simulink model "VCU_Modes"  (R2025b)
settings: Solver=FixedStepDiscrete  StartTime=0.0  StopTime=10.0  FixedStep=0.01  RelTol=1e-3
values from neighbouring files (symbols this model uses):
  c_VCU_BattCurrDrvThd = 100.0    [VCU_Modes.sldd]
  c_VCU_BattCurrDrvTime = 200.0    [VCU_Modes.sldd]
  c_VCU_BattCurrParkThd = 5.0    [VCU_Modes.sldd]
  c_VCU_BattCurrPeakDrvThd = 180.0    [VCU_Modes.sldd]
  c_VCU_BattSocDrvThd = 10.0    [VCU_Modes.sldd]
  c_VCU_BattSocLimpThd = 5.0    [VCU_Modes.sldd]
  c_VCU_BattTempDrvThdMax = 60.0    [VCU_Modes.sldd]
  c_VCU_BattTempParkThd = 45.0    [VCU_Modes.sldd]
  c_VCU_BattTempParkThdFlt = 55.0    [VCU_Modes.sldd]
  c_VCU_DrvThdWait = 100.0    [VCU_Modes.sldd]
  c_VCU_EcuTempDrvThdMax = 95.0    [VCU_Modes.sldd]
  c_VCU_EcuTempParkThd = 70.0    [VCU_Modes.sldd]
  c_VCU_EcuTempParkThdFlt = 85.0    [VCU_Modes.sldd]
  c_VCU_FailSafeThdTime = 200.0    [VCU_Modes.sldd]
  c_VCU_FrontLampExclusive_B = 0.0    [VCU_Modes.sldd]
  c_VCU_HeadLampAmbientThd = 300.0    [VCU_Modes.sldd]
  c_VCU_HeadlampAutoEnable_B = 1.0    [VCU_Modes.sldd]
  c_VCU_HeadlampManualOverride_B = 1.0    [VCU_Modes.sldd]
  c_VCU_LongPressTimeThd = 200.0    [VCU_Modes.sldd]
  c_VCU_MotTempDrvThdMax = 120.0    [VCU_Modes.sldd]
  c_VCU_MotTempParkThd = 80.0    [VCU_Modes.sldd]
  c_VCU_MotTempParkThdFlt = 100.0    [VCU_Modes.sldd]
  c_VCU_ParkExtThdWait = 100.0    [VCU_Modes.sldd]
  c_VCU_ParkThdWait = 100.0    [VCU_Modes.sldd]
  F32_ZERO = 0.0    [VCU_Modes.sldd]
  FALSE = 0.0    [VCU_Modes.sldd]
  TRUE = 1.0    [VCU_Modes.sldd]
  UI8_ZERO = 0.0    [VCU_Modes.sldd]
undefined symbols (not defined in the file or in its folder): POWER_MODE, SIG_STATUS, VCU_MODE
libraries: Sanu_Lib x9, simulink x1
(part 1 of 2)
Description:
  | Different types of VCU modes and Drive modes control.
  | Based on VCU and Drive modes vehicle performance.
settings Model: DataDictionary=VCU_Modes.sldd  Creator=2503-00091  LastModifiedBy=2503-00091
settings OptimizationCC: DefaultParameterBehavior=Inlined  EnhancedBackFolding=on  PassReuseOutputArgsAs=Individual arguments  ZeroExternalMemoryAtStartup=off  ZeroInternalMemoryAtStartup=off  OptimizeBlockOrder=speed  DifferentSizesBufferReuse=on  OptimizationCustomize=off  LabelGuidedReuse=on  EfficientTunableParamExpr=on
settings DebuggingCC: AlgebraicLoopMsg=error  ArtificialAlgebraicLoopMsg=error  ParameterTunabilityLossMsg=error  UnitsInconsistencyMsg=none
settings SFSimCC: MATLABDynamicMemAlloc=off
settings RTWCC: SystemTargetFile=ert.tlc  TemplateMakefile=ert_default_tmf  Description=Embedded Coder
settings CodeAppCC: ForceParamTrailComments=on  IgnoreCustomStorageClasses=off  OperatorAnnotations=on  SimulinkDataObjDesc=on  SFDataObjDesc=on  MATLABFcnDesc=on  CustomSymbolStrFcnArg=$I$N$M  CustomSymbolStrBlkIO=$N$M  InsertBlockDesc=on
settings ERTTargetCC: ERTCustomFileTemplate=example_file_process.tlc  TargetLangStandard=C99 (ISO)  GenerateSampleERTMain=on  LogVarNameModifier=none

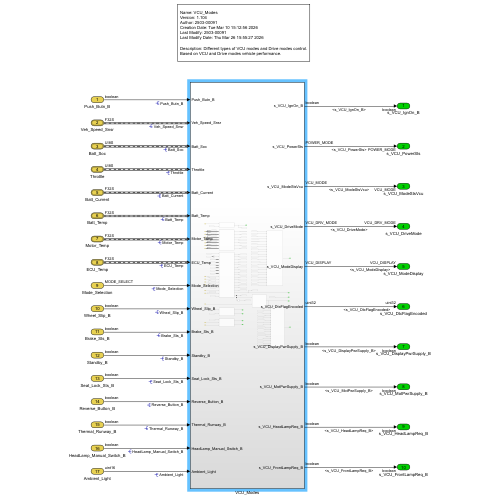
[thumbnail: Simulink's stored preview of the top-level diagram]
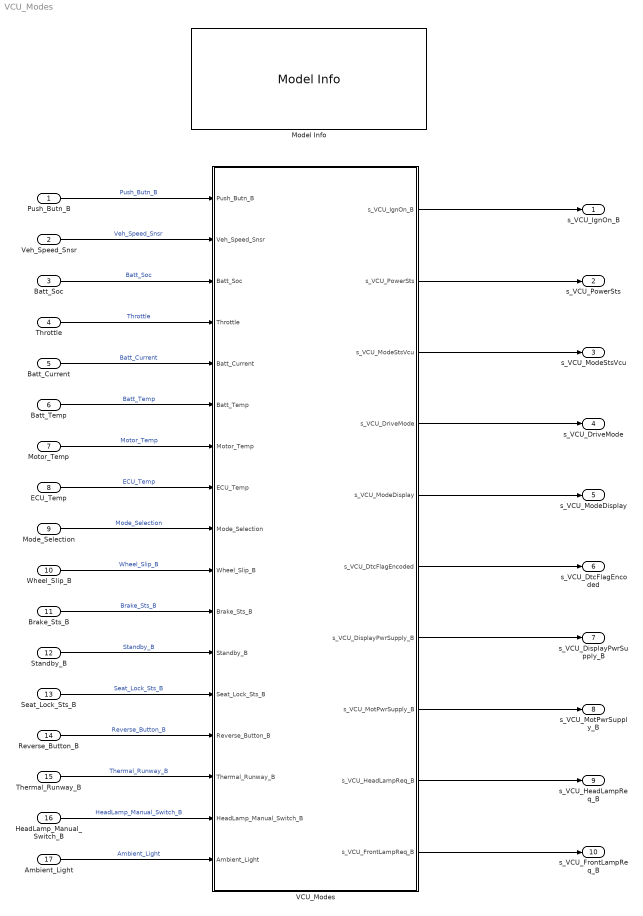
== system VCU_Modes ==
  Push_Butn_B : Inport  OutDataTypeStr=boolean  PortDimensions=1
  Veh_Speed_Snsr : Inport  Port=2  OutDataTypeStr=Bus: F32S  PortDimensions=1  BusOutputAsStruct=on
  Batt_Soc : Inport  Port=3  OutDataTypeStr=Bus: UI8S  PortDimensions=1  BusOutputAsStruct=on
  Throttle : Inport  Port=4  OutDataTypeStr=Bus: UI8S  PortDimensions=1  BusOutputAsStruct=on
  Batt_Current : Inport  Port=5  OutDataTypeStr=Bus: F32S  PortDimensions=1  BusOutputAsStruct=on
  Batt_Temp : Inport  Port=6  OutDataTypeStr=Bus: F32S  PortDimensions=1  BusOutputAsStruct=on
  Motor_Temp : Inport  Port=7  OutDataTypeStr=Bus: F32S  PortDimensions=1  BusOutputAsStruct=on
  ECU_Temp : Inport  Port=8  OutDataTypeStr=Bus: F32S  PortDimensions=1  BusOutputAsStruct=on
  Mode_Selection : Inport  Port=9  OutDataTypeStr=Enum: MODE_SELECT  PortDimensions=1
  Wheel_Slip_B : Inport  Port=10  OutDataTypeStr=boolean  PortDimensions=1
  Brake_Sts_B : Inport  Port=11  OutDataTypeStr=boolean  PortDimensions=1
  Standby_B : Inport  Port=12  OutDataTypeStr=boolean  PortDimensions=1
  Seat_Lock_Sts_B : Inport  Port=13  OutDataTypeStr=boolean  PortDimensions=1
  Reverse_Button_B : Inport  Port=14  OutDataTypeStr=boolean  PortDimensions=1
  Thermal_Runway_B : Inport  Port=15  OutDataTypeStr=boolean  PortDimensions=1
  HeadLamp_Manual_Switch_B : Inport  Port=16  OutDataTypeStr=boolean  PortDimensions=1
  Ambient_Light : Inport  Port=17  OutDataTypeStr=uint16  PortDimensions=1
  Model Info : simulink/Model-Wide Utilities/Model Info  Frame=on  DisplayStringWithTags=|  HorizontalTextAlignment=Left  LeftAlignmentValue=0.02
      | Name: %<ModelName>
      | Version: %<ModelVersion>
      | Author: %<Creator>
      | Creation Date: %<Created>
      | Last Modify: %<LastModifiedBy>
      | Last Modify Date: %<LastModificationDate>
      | 
      | Description: %<Description>
  VCU_Modes : Subsystem
  s_VCU_IgnOn_B : Outport  OutDataTypeStr=boolean  PortDimensions=1
  s_VCU_PowerSts : Outport  Port=2  OutDataTypeStr=Enum: POWER_MODE  PortDimensions=1
  s_VCU_ModeStsVcu : Outport  Port=3  OutDataTypeStr=Enum: VCU_MODE  PortDimensions=1
  s_VCU_DriveMode : Outport  Port=4  OutDataTypeStr=Enum: VCU_DRV_MODE  PortDimensions=1
  s_VCU_ModeDisplay : Outport  Port=5  OutDataTypeStr=Enum: VCU_DISPLAY  PortDimensions=1
  s_VCU_DtcFlagEncoded : Outport  Port=6  OutDataTypeStr=uint32  PortDimensions=1
  s_VCU_DisplayPwrSupply_B : Outport  Port=7  OutDataTypeStr=boolean  PortDimensions=1
  s_VCU_MotPwrSupply_B : Outport  Port=8  OutDataTypeStr=boolean  PortDimensions=1
  s_VCU_HeadLampReq_B : Outport  Port=9  OutDataTypeStr=boolean  PortDimensions=1
  s_VCU_FrontLampReq_B : Outport  Port=10  OutDataTypeStr=boolean  PortDimensions=1
  wires:
  Push_Butn_B/1 -> VCU_Modes/1(Push_Butn_B)  "Push_Butn_B"
  Veh_Speed_Snsr/1 -> VCU_Modes/2(Veh_Speed_Snsr)  "Veh_Speed_Snsr"
  Batt_Soc/1 -> VCU_Modes/3(Batt_Soc)  "Batt_Soc"
  Throttle/1 -> VCU_Modes/4(Throttle)  "Throttle"
  ECU_Temp/1 -> VCU_Modes/8(ECU_Temp)  "ECU_Temp"
  Batt_Current/1 -> VCU_Modes/5(Batt_Current)  "Batt_Current"
  Batt_Temp/1 -> VCU_Modes/6(Batt_Temp)  "Batt_Temp"
  Motor_Temp/1 -> VCU_Modes/7(Motor_Temp)  "Motor_Temp"
  Mode_Selection/1 -> VCU_Modes/9(Mode_Selection)  "Mode_Selection"
  Wheel_Slip_B/1 -> VCU_Modes/10(Wheel_Slip_B)  "Wheel_Slip_B"
  Brake_Sts_B/1 -> VCU_Modes/11(Brake_Sts_B)  "Brake_Sts_B"
  Standby_B/1 -> VCU_Modes/12(Standby_B)  "Standby_B"
  Seat_Lock_Sts_B/1 -> VCU_Modes/13(Seat_Lock_Sts_B)  "Seat_Lock_Sts_B"
  Reverse_Button_B/1 -> VCU_Modes/14(Reverse_Button_B)  "Reverse_Button_B"
  Thermal_Runway_B/1 -> VCU_Modes/15(Thermal_Runway_B)  "Thermal_Runway_B"
  VCU_Modes/2(s_VCU_PowerSts) -> s_VCU_PowerSts/1
  VCU_Modes/3(s_VCU_ModeStsVcu) -> s_VCU_ModeStsVcu/1
  VCU_Modes/6(s_VCU_DtcFlagEncoded) -> s_VCU_DtcFlagEncoded/1
  VCU_Modes/5(s_VCU_ModeDisplay) -> s_VCU_ModeDisplay/1
  VCU_Modes/4(s_VCU_DriveMode) -> s_VCU_DriveMode/1
  HeadLamp_Manual_Switch_B/1 -> VCU_Modes/16(HeadLamp_Manual_Switch_B)  "HeadLamp_Manual_Switch_B"
  Ambient_Light/1 -> VCU_Modes/17(Ambient_Light)  "Ambient_Light"
  VCU_Modes/7(s_VCU_DisplayPwrSupply_B) -> s_VCU_DisplayPwrSupply_B/1
  VCU_Modes/9(s_VCU_HeadLampReq_B) -> s_VCU_HeadLampReq_B/1
  VCU_Modes/8(s_VCU_MotPwrSupply_B) -> s_VCU_MotPwrSupply_B/1
  VCU_Modes/10(s_VCU_FrontLampReq_B) -> s_VCU_FrontLampReq_B/1
  VCU_Modes/1(s_VCU_IgnOn_B) -> s_VCU_IgnOn_B/1

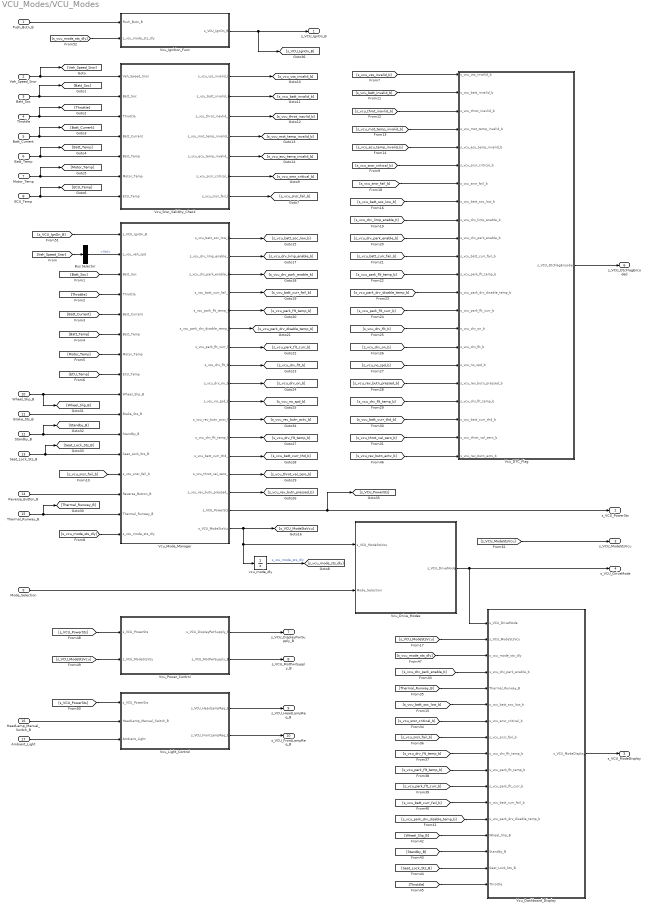
== system VCU_Modes/VCU_Modes ==
  Push_Butn_B : Inport
  Veh_Speed_Snsr : Inport  Port=2
  Batt_Soc : Inport  Port=3
  Throttle : Inport  Port=4
  Batt_Current : Inport  Port=5
  Batt_Temp : Inport  Port=6
  Motor_Temp : Inport  Port=7
  ECU_Temp : Inport  Port=8
  Mode_Selection : Inport  Port=9
  Wheel_Slip_B : Inport  Port=10
  Brake_Sts_B : Inport  Port=11
  Standby_B : Inport  Port=12
  Seat_Lock_Sts_B : Inport  Port=13
  Reverse_Button_B : Inport  Port=14
  Thermal_Runway_B : Inport  Port=15
  HeadLamp_Manual_Switch_B : Inport  Port=16
  Ambient_Light : Inport  Port=17
  Bus Selector : BusSelector  OutputSignals=Val
  Vcu_DTC_Flag : Subsystem  TreatAsAtomicUnit=on  RTWFcnName=Vcu_DTC_Flag
      settings: RTWSystemCode=Nonreusable function  RTWFcnNameOpts=User specified
  Vcu_Dashboard_Display : Subsystem  TreatAsAtomicUnit=on  RTWFcnName=Vcu_Dashboard_Display
      settings: RTWSystemCode=Nonreusable function  RTWFcnNameOpts=User specified
  Vcu_Drive_Modes : Subsystem  TreatAsAtomicUnit=on  RTWFcnName=Vcu_Drive_Modes
      settings: RTWSystemCode=Nonreusable function  RTWFcnNameOpts=User specified
  Vcu_Ignition_Func : Subsystem  TreatAsAtomicUnit=on  RTWFcnName=Vcu_Ignition_Func
      settings: RTWSystemCode=Nonreusable function  RTWFcnNameOpts=User specified
  Vcu_Light_Control : Subsystem  TreatAsAtomicUnit=on  RTWFcnName=Vcu_Light_Control
      settings: RTWSystemCode=Nonreusable function  RTWFcnNameOpts=User specified
  Vcu_Mode_Manager : Subsystem  TreatAsAtomicUnit=on  RTWFcnName=Vcu_Mode_Manager
      settings: RTWSystemCode=Nonreusable function  RTWFcnNameOpts=User specified
  Vcu_Power_Control : Subsystem  TreatAsAtomicUnit=on  RTWFcnName=Vcu_Power_Control
      settings: RTWSystemCode=Nonreusable function  RTWFcnNameOpts=User specified
  Vcu_Snsr_Validity_Check : Subsystem  TreatAsAtomicUnit=on  RTWFcnName=Vcu_Snsr_Validity_Check
      settings: RTWSystemCode=Nonreusable function  RTWFcnNameOpts=User specified
  vcu_mode_dly : UnitDelay  InitialCondition=VCU_MODE.VCU_PWR_OFF  SampleTime=-1  HasFrameUpgradeWarning=on
      settings: AttributesFormatString=Init: %<InitialCondition>
  s_VCU_IgnOn_B : Outport
  s_VCU_PowerSts : Outport  Port=2
  s_VCU_ModeStsVcu : Outport  Port=3
  s_VCU_DriveMode : Outport  Port=4
  s_VCU_ModeDisplay : Outport  Port=5
  s_VCU_DtcFlagEncoded : Outport  Port=6
  s_VCU_DisplayPwrSupply_B : Outport  Port=7
  s_VCU_MotPwrSupply_B : Outport  Port=8
  s_VCU_HeadLampReq_B : Outport  Port=9
  s_VCU_FrontLampReq_B : Outport  Port=10
  wires:
  Veh_Speed_Snsr/1 -> Vcu_Snsr_Validity_Check/1(Veh_Speed_Snsr), [Veh_Speed_Snsr]
  Motor_Temp/1 -> Vcu_Snsr_Validity_Check/6(Motor_Temp), [Motor_Temp]
  Batt_Temp/1 -> Vcu_Snsr_Validity_Check/5(Batt_Temp), [Batt_Temp]
  Batt_Current/1 -> Vcu_Snsr_Validity_Check/4(Batt_Current), [Batt_Current]
  Throttle/1 -> Vcu_Snsr_Validity_Check/3(Throttle), [Throttle]
  ECU_Temp/1 -> Vcu_Snsr_Validity_Check/7(ECU_Temp), [ECU_Temp]
  Batt_Soc/1 -> Vcu_Snsr_Validity_Check/2(Batt_Soc), [Batt_Soc]
  [Veh_Speed_Snsr] -> Bus Selector/1
  Push_Butn_B/1 -> Vcu_Ignition_Func/1(Push_Butn_B)
  [Batt_Soc] -> Vcu_Mode_Manager/3(Batt_Soc)
  [Throttle] -> Vcu_Mode_Manager/4(Throttle)
  [Batt_Current] -> Vcu_Mode_Manager/5(Batt_Current)
  [Batt_Temp] -> Vcu_Mode_Manager/6(Batt_Temp)
  [Motor_Temp] -> Vcu_Mode_Manager/7(Motor_Temp)
  [ECU_Temp] -> Vcu_Mode_Manager/8(ECU_Temp)
  Wheel_Slip_B/1 -> [Wheel_Slip_B], Vcu_Mode_Manager/9(Wheel_Slip_B)
  Brake_Sts_B/1 -> Vcu_Mode_Manager/10(Brake_Sts_B)
  Standby_B/1 -> [Standby_B], Vcu_Mode_Manager/11(Standby_B)
  Seat_Lock_Sts_B/1 -> [Seat_Lock_Sts_B], Vcu_Mode_Manager/12(Seat_Lock_Sts_B)
  Reverse_Button_B/1 -> Vcu_Mode_Manager/14(Reverse_Button_B)
  Thermal_Runway_B/1 -> [Thermal_Runway_B], Vcu_Mode_Manager/15(Thermal_Runway_B)
  [s_vcu_snsr_fail_b] -> Vcu_Mode_Manager/13(s_vcu_snsr_fail_b)
  vcu_mode_dly/1 -> [s_vcu_mode_sts_dly]  "s_vcu_mode_sts_dly"
  [s_vcu_mode_sts_dly] -> Vcu_Mode_Manager/16(s_vcu_mode_sts_dly)
  Mode_Selection/1 -> Vcu_Drive_Modes/2(Mode_Selection)
  Vcu_Mode_Manager/17(s_VCU_ModeStsVcu) -> Vcu_Drive_Modes/1(s_VCU_ModeStsVcu), vcu_mode_dly/1, [s_VCU_ModeStsVcu]
  Vcu_Drive_Modes/1(s_VCU_DriveMode) -> s_VCU_DriveMode/1, Vcu_Dashboard_Display/1(s_VCU_DriveMode)
  Vcu_Snsr_Validity_Check/6(s_vcu_snsr_critical_b) -> [s_vcu_snsr_critical_b]
  Vcu_Snsr_Validity_Check/7(s_vcu_snsr_fail_b) -> [s_vcu_snsr_fail_b]
  Vcu_Snsr_Validity_Check/1(s_vcu_vss_invalid_b) -> [s_vcu_vss_invalid_b]
  Vcu_Snsr_Validity_Check/4(s_vcu_mot_temp_invalid_b) -> [s_vcu_mot_temp_invalid_b]
  Vcu_Snsr_Validity_Check/3(s_vcu_throt_inavlid_b) -> [s_vcu_throt_inavlid_b]
  Vcu_Snsr_Validity_Check/2(s_vcu_batt_invalid_b) -> [s_vcu_batt_invalid_b]
  Vcu_Snsr_Validity_Check/5(s_vcu_ecu_temp_invalid_b) -> [s_vcu_ecu_temp_invalid_b]
  [s_vcu_vss_invalid_b] -> Vcu_DTC_Flag/1(s_vcu_vss_invalid_b)
  [s_vcu_batt_invalid_b] -> Vcu_DTC_Flag/2(s_vcu_batt_invalid_b)
  [s_vcu_throt_inavlid_b] -> Vcu_DTC_Flag/3(s_vcu_throt_inavlid_b)
  [s_vcu_mot_temp_invalid_b] -> Vcu_DTC_Flag/4(s_vcu_mot_temp_invalid_b)
  [s_vcu_ecu_temp_invalid_b] -> Vcu_DTC_Flag/5(s_vcu_ecu_temp_invalid_b)
  [s_vcu_snsr_critical_b] -> Vcu_DTC_Flag/6(s_vcu_snsr_critical_b)
  Vcu_Dashboard_Display/1(s_VCU_ModeDisplay) -> s_VCU_ModeDisplay/1
  Vcu_Mode_Manager/1(s_vcu_batt_soc_low_b) -> [s_vcu_batt_soc_low_b]
  [s_vcu_batt_soc_low_b] -> Vcu_Dashboard_Display/6(s_vcu_batt_soc_low_b)
  [s_vcu_batt_soc_low_b] -> Vcu_DTC_Flag/8(s_vcu_batt_soc_low_b)
  [s_VCU_ModeStsVcu] -> Vcu_Dashboard_Display/2(s_VCU_ModeStsVcu)
  [s_vcu_snsr_fail_b] -> Vcu_DTC_Flag/7(s_vcu_snsr_fail_b)
  Vcu_Mode_Manager/2(s_vcu_drv_limp_enable_b) -> [s_vcu_drv_limp_enable_b]
  [s_vcu_drv_limp_enable_b] -> Vcu_DTC_Flag/9(s_vcu_drv_limp_enable_b)
  Vcu_Mode_Manager/3(s_vcu_drv_park_enable_b) -> [s_vcu_drv_park_enable_b]
  [s_vcu_drv_park_enable_b] -> Vcu_DTC_Flag/10(s_vcu_drv_park_enable_b)
  Vcu_Mode_Manager/4(s_vcu_batt_curr_fail_b) -> [s_vcu_batt_curr_fail_b]
  [s_vcu_batt_curr_fail_b] -> Vcu_DTC_Flag/11(s_vcu_batt_curr_fail_b)
  Vcu_Mode_Manager/5(s_vcu_park_flt_temp_b) -> [s_vcu_park_flt_temp_b]
  [s_vcu_park_flt_temp_b] -> Vcu_DTC_Flag/12(s_vcu_park_flt_temp_b)
  Vcu_Mode_Manager/6(s_vcu_park_drv_disable_temp_b) -> [s_vcu_park_drv_disable_temp_b]
  [s_vcu_park_drv_disable_temp_b] -> Vcu_DTC_Flag/13(s_vcu_park_drv_disable_temp_b)
  Vcu_Mode_Manager/7(s_vcu_park_flt_curr_b) -> [s_vcu_park_flt_curr_b]
  [s_vcu_park_flt_curr_b] -> Vcu_DTC_Flag/14(s_vcu_park_flt_curr_b)
  Vcu_Mode_Manager/8(s_vcu_drv_flt_b) -> [s_vcu_drv_flt_b]
  [s_vcu_drv_flt_b] -> Vcu_DTC_Flag/15(s_vcu_drv_on_b)
  Vcu_Mode_Manager/9(s_vcu_drv_on_b) -> [s_vcu_drv_on_b]
  [s_vcu_drv_on_b] -> Vcu_DTC_Flag/16(s_vcu_drv_flt_b)
  Vcu_Mode_Manager/10(s_vcu_no_spd_b) -> [s_vcu_no_spd_b]
  [s_vcu_no_spd_b] -> Vcu_DTC_Flag/17(s_vcu_no_spd_b)
  Vcu_Mode_Manager/15(s_vcu_rev_butn_pressed_b) -> [s_vcu_rev_butn_pressed_b]
  [s_vcu_rev_butn_pressed_b] -> Vcu_DTC_Flag/18(s_vcu_rev_butn_pressed_b)
  Vcu_Mode_Manager/12(s_vcu_drv_flt_temp_b) -> [s_vcu_drv_flt_temp_b]
  [s_vcu_drv_flt_temp_b] -> Vcu_DTC_Flag/19(s_vcu_drv_flt_temp_b)
  Vcu_Mode_Manager/13(s_vcu_batt_curr_thd_b) -> [s_vcu_batt_curr_thd_b]
  [s_vcu_batt_curr_thd_b] -> Vcu_DTC_Flag/20(s_vcu_batt_curr_thd_b)
  Vcu_Mode_Manager/14(s_vcu_throt_val_zero_b) -> [s_vcu_throt_val_zero_b]
  [s_vcu_throt_val_zero_b] -> Vcu_DTC_Flag/21(s_vcu_throt_val_zero_b)
  Vcu_Mode_Manager/16(s_VCU_PowerSts) -> [s_VCU_PowerSts], s_VCU_PowerSts/1
  [s_VCU_ModeStsVcu] -> s_VCU_ModeStsVcu/1
  Vcu_DTC_Flag/1(s_VCU_DtcFlagEncoded) -> s_VCU_DtcFlagEncoded/1
  [s_vcu_drv_park_enable_b] -> Vcu_Dashboard_Display/4(s_vcu_drv_park_enable_b)
  [Thermal_Runway_B] -> Vcu_Dashboard_Display/5(Thermal_Runway_B)
  [s_vcu_snsr_critical_b] -> Vcu_Dashboard_Display/7(s_vcu_snsr_critical_b)
  [s_vcu_snsr_fail_b] -> Vcu_Dashboard_Display/8(s_vcu_snsr_fail_b)
  [s_vcu_drv_flt_temp_b] -> Vcu_Dashboard_Display/9(s_vcu_drv_flt_temp_b)
  [s_vcu_park_flt_temp_b] -> Vcu_Dashboard_Display/10(s_vcu_park_flt_temp_b)
  [s_vcu_park_flt_curr_b] -> Vcu_Dashboard_Display/11(s_vcu_park_flt_curr_b)
  [s_vcu_batt_curr_fail_b] -> Vcu_Dashboard_Display/12(s_vcu_batt_curr_fail_b)
  [s_vcu_park_drv_disable_temp_b] -> Vcu_Dashboard_Display/13(s_vcu_park_drv_disable_temp_b)
  [Wheel_Slip_B] -> Vcu_Dashboard_Display/14(Wheel_Slip_B)
  [Standby_B] -> Vcu_Dashboard_Display/15(Standby_B)
  [Throttle] -> Vcu_Dashboard_Display/17(Throttle)
  [Seat_Lock_Sts_B] -> Vcu_Dashboard_Display/16(Seat_Lock_Sts_B)
  Bus Selector/1 -> Vcu_Mode_Manager/2(s_vcu_veh_spd)  "<Val>"
  Vcu_Mode_Manager/11(s_vcu_rev_butn_actv_b) -> [s_vcu_rev_butn_actv_b]
  [s_vcu_rev_butn_actv_b] -> Vcu_DTC_Flag/22(s_vcu_rev_butn_actv_b)
  [s_vcu_mode_sts_dly] -> Vcu_Dashboard_Display/3(s_vcu_mode_sts_dly)
  [s_VCU_PowerSts] -> Vcu_Power_Control/1(s_VCU_PowerSts)
  [s_VCU_ModeStsVcu] -> Vcu_Power_Control/2("s_VCU_ModeStsVcu ")
  [s_VCU_PowerSts] -> Vcu_Light_Control/1(s_VCU_PowerSts)
  HeadLamp_Manual_Switch_B/1 -> Vcu_Light_Control/2(HeadLamp_Manual_Switch_B)
  Ambient_Light/1 -> Vcu_Light_Control/3(Ambient_Light)
  Vcu_Power_Control/1(s_VCU_DisplayPwrSupply_B) -> s_VCU_DisplayPwrSupply_B/1
  Vcu_Power_Control/2(s_VCU_MotPwrSupply_B) -> s_VCU_MotPwrSupply_B/1
  Vcu_Light_Control/1(s_VCU_HeadLampReq_B) -> s_VCU_HeadLampReq_B/1
  Vcu_Light_Control/2(s_VCU_FrontLampReq_B) -> s_VCU_FrontLampReq_B/1
  [s_VCU_IgnOn_B] -> Vcu_Mode_Manager/1(s_VCU_IgnOn_B)
  Vcu_Ignition_Func/1(s_VCU_IgnOn_B) -> [s_VCU_IgnOn_B], s_VCU_IgnOn_B/1
  [s_vcu_mode_sts_dly] -> Vcu_Ignition_Func/2(s_vcu_mode_sts_dly)

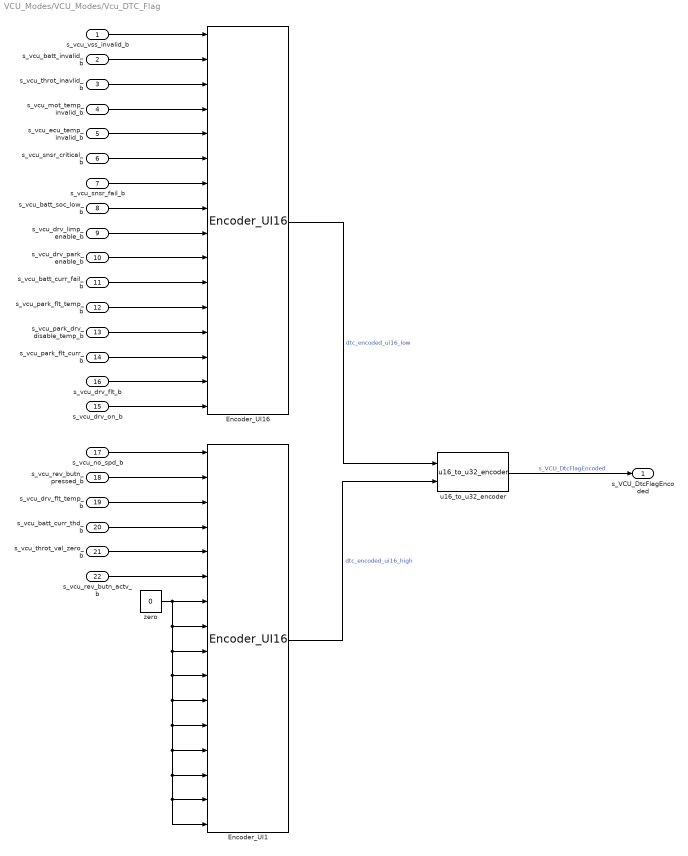
== system VCU_Modes/VCU_Modes/Vcu_DTC_Flag ==
  s_vcu_vss_invalid_b : Inport
  s_vcu_batt_invalid_b : Inport  Port=2
  s_vcu_throt_inavlid_b : Inport  Port=3
  s_vcu_mot_temp_invalid_b : Inport  Port=4
  s_vcu_ecu_temp_invalid_b : Inport  Port=5
  s_vcu_snsr_critical_b : Inport  Port=6
  s_vcu_snsr_fail_b : Inport  Port=7
  s_vcu_batt_soc_low_b : Inport  Port=8
  s_vcu_drv_limp_enable_b : Inport  Port=9
  s_vcu_drv_park_enable_b : Inport  Port=10
  s_vcu_batt_curr_fail_b : Inport  Port=11
  s_vcu_park_flt_temp_b : Inport  Port=12
  s_vcu_park_drv_disable_temp_b : Inport  Port=13
  s_vcu_park_flt_curr_b : Inport  Port=14
  s_vcu_drv_on_b : Inport  Port=15
  s_vcu_drv_flt_b : Inport  Port=16
  s_vcu_no_spd_b : Inport  Port=17
  s_vcu_rev_butn_pressed_b : Inport  Port=18
  s_vcu_drv_flt_temp_b : Inport  Port=19
  s_vcu_batt_curr_thd_b : Inport  Port=20
  s_vcu_throt_val_zero_b : Inport  Port=21
  s_vcu_rev_butn_actv_b : Inport  Port=22
  Encoder_UI1 : Sanu_Lib/Encoder_UI16  SystemSampleTime=-1  VariantActivationTime=update diagram  EmptyChoice=off  PassThrough=off  PassThroughVariantControl=(default)  EmptyChoiceVariantControl=(default)  AllowFlexibleInterface=on  Latency=0  AutoFrameSizeCalculation=off
  Encoder_UI16 : Sanu_Lib/Encoder_UI16  SystemSampleTime=-1  VariantActivationTime=update diagram  EmptyChoice=off  PassThrough=off  PassThroughVariantControl=(default)  EmptyChoiceVariantControl=(default)  AllowFlexibleInterface=on  Latency=0  AutoFrameSizeCalculation=off
  u16_to_u32_encoder : Sanu_Lib/u16_to_u32_encoder  SystemSampleTime=-1  VariantActivationTime=update diagram  EmptyChoice=off  PassThrough=off  PassThroughVariantControl=(default)  EmptyChoiceVariantControl=(default)  AllowFlexibleInterface=on  Latency=0  AutoFrameSizeCalculation=off
  zero : Constant  Value=0  OutDataTypeStr=boolean  SampleTime=-1
  s_VCU_DtcFlagEncoded : Outport
  wires:
  s_vcu_vss_invalid_b/1 -> Encoder_UI16/1
  s_vcu_batt_invalid_b/1 -> Encoder_UI16/2
  s_vcu_throt_inavlid_b/1 -> Encoder_UI16/3
  s_vcu_mot_temp_invalid_b/1 -> Encoder_UI16/4
  s_vcu_ecu_temp_invalid_b/1 -> Encoder_UI16/5
  s_vcu_snsr_critical_b/1 -> Encoder_UI16/6
  s_vcu_snsr_fail_b/1 -> Encoder_UI16/7
  s_vcu_batt_soc_low_b/1 -> Encoder_UI16/8
  s_vcu_drv_limp_enable_b/1 -> Encoder_UI16/9
  s_vcu_drv_park_enable_b/1 -> Encoder_UI16/10
  s_vcu_batt_curr_fail_b/1 -> Encoder_UI16/11
  s_vcu_park_flt_temp_b/1 -> Encoder_UI16/12
  s_vcu_park_drv_disable_temp_b/1 -> Encoder_UI16/13
  s_vcu_park_flt_curr_b/1 -> Encoder_UI16/14
  s_vcu_drv_flt_b/1 -> Encoder_UI16/15
  s_vcu_drv_on_b/1 -> Encoder_UI16/16
  Encoder_UI16/1 -> u16_to_u32_encoder/1  "dtc_encoded_ui16_low"
  Encoder_UI1/1 -> u16_to_u32_encoder/2  "dtc_encoded_ui16_high"
  u16_to_u32_encoder/1 -> s_VCU_DtcFlagEncoded/1  "s_VCU_DtcFlagEncoded"
  s_vcu_no_spd_b/1 -> Encoder_UI1/1
  s_vcu_rev_butn_pressed_b/1 -> Encoder_UI1/2
  s_vcu_drv_flt_temp_b/1 -> Encoder_UI1/3
  s_vcu_batt_curr_thd_b/1 -> Encoder_UI1/4
  s_vcu_throt_val_zero_b/1 -> Encoder_UI1/5
  zero/1 -> Encoder_UI1/7, Encoder_UI1/8, Encoder_UI1/9, Encoder_UI1/10, Encoder_UI1/11, Encoder_UI1/12, Encoder_UI1/13, Encoder_UI1/14, Encoder_UI1/15, Encoder_UI1/16
  s_vcu_rev_butn_actv_b/1 -> Encoder_UI1/6

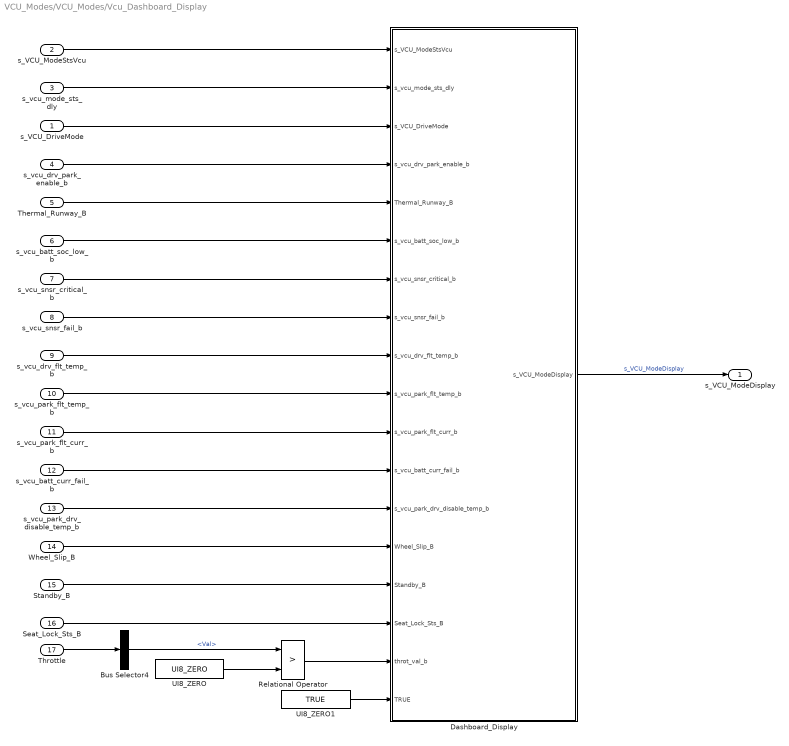
== system VCU_Modes/VCU_Modes/Vcu_Dashboard_Display ==
  s_VCU_DriveMode : Inport
  s_VCU_ModeStsVcu : Inport  Port=2
  s_vcu_mode_sts_dly : Inport  Port=3
  s_vcu_drv_park_enable_b : Inport  Port=4
  Thermal_Runway_B : Inport  Port=5
  s_vcu_batt_soc_low_b : Inport  Port=6
  s_vcu_snsr_critical_b : Inport  Port=7
  s_vcu_snsr_fail_b : Inport  Port=8
  s_vcu_drv_flt_temp_b : Inport  Port=9
  s_vcu_park_flt_temp_b : Inport  Port=10
  s_vcu_park_flt_curr_b : Inport  Port=11
  s_vcu_batt_curr_fail_b : Inport  Port=12
  s_vcu_park_drv_disable_temp_b : Inport  Port=13
  Wheel_Slip_B : Inport  Port=14
  Standby_B : Inport  Port=15
  Seat_Lock_Sts_B : Inport  Port=16
  Throttle : Inport  Port=17
  Bus Selector4 : BusSelector  OutputSignals=Val
  Dashboard_Display : Stateflow chart  TreatAsAtomicUnit=on
  Relational Operator : RelationalOperator  Operator=>  OutDataTypeStr=boolean  RndMeth=Simplest  InputSameDT=off
  UI8_ZERO : Constant  Value=UI8_ZERO  OutDataTypeStr=uint8  SampleTime=-1
  UI8_ZERO1 : Constant  Value=TRUE  OutDataTypeStr=boolean  SampleTime=-1
  s_VCU_ModeDisplay : Outport
  wires:
  s_VCU_ModeStsVcu/1 -> Dashboard_Display/1(s_VCU_ModeStsVcu)
  Bus Selector4/1 -> Relational Operator/1  "<Val>"
  Throttle/1 -> Bus Selector4/1
  Standby_B/1 -> Dashboard_Display/15(Standby_B)
  s_vcu_park_flt_temp_b/1 -> Dashboard_Display/10(s_vcu_park_flt_temp_b)
  Wheel_Slip_B/1 -> Dashboard_Display/14(Wheel_Slip_B)
  UI8_ZERO/1 -> Relational Operator/2
  s_VCU_DriveMode/1 -> Dashboard_Display/3(s_VCU_DriveMode)
  s_vcu_drv_park_enable_b/1 -> Dashboard_Display/4(s_vcu_drv_park_enable_b)
  Thermal_Runway_B/1 -> Dashboard_Display/5(Thermal_Runway_B)
  s_vcu_batt_soc_low_b/1 -> Dashboard_Display/6(s_vcu_batt_soc_low_b)
  s_vcu_snsr_critical_b/1 -> Dashboard_Display/7(s_vcu_snsr_critical_b)
  s_vcu_snsr_fail_b/1 -> Dashboard_Display/8(s_vcu_snsr_fail_b)
  s_vcu_drv_flt_temp_b/1 -> Dashboard_Display/9(s_vcu_drv_flt_temp_b)
  s_vcu_park_flt_curr_b/1 -> Dashboard_Display/11(s_vcu_park_flt_curr_b)
  s_vcu_batt_curr_fail_b/1 -> Dashboard_Display/12(s_vcu_batt_curr_fail_b)
  s_vcu_park_drv_disable_temp_b/1 -> Dashboard_Display/13(s_vcu_park_drv_disable_temp_b)
  Seat_Lock_Sts_B/1 -> Dashboard_Display/16(Seat_Lock_Sts_B)
  Relational Operator/1 -> Dashboard_Display/17(throt_val_b)
  Dashboard_Display/1(s_VCU_ModeDisplay) -> s_VCU_ModeDisplay/1  "s_VCU_ModeDisplay"
  UI8_ZERO1/1 -> Dashboard_Display/18(TRUE)
  s_vcu_mode_sts_dly/1 -> Dashboard_Display/2(s_vcu_mode_sts_dly)

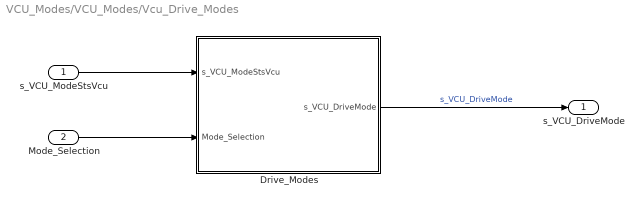
== system VCU_Modes/VCU_Modes/Vcu_Drive_Modes ==
  s_VCU_ModeStsVcu : Inport
  Mode_Selection : Inport  Port=2
  Drive_Modes : Stateflow chart  TreatAsAtomicUnit=on
  s_VCU_DriveMode : Outport
  wires:
  Mode_Selection/1 -> Drive_Modes/2(Mode_Selection)
  Drive_Modes/1(s_VCU_DriveMode) -> s_VCU_DriveMode/1  "s_VCU_DriveMode"
  s_VCU_ModeStsVcu/1 -> Drive_Modes/1(s_VCU_ModeStsVcu)

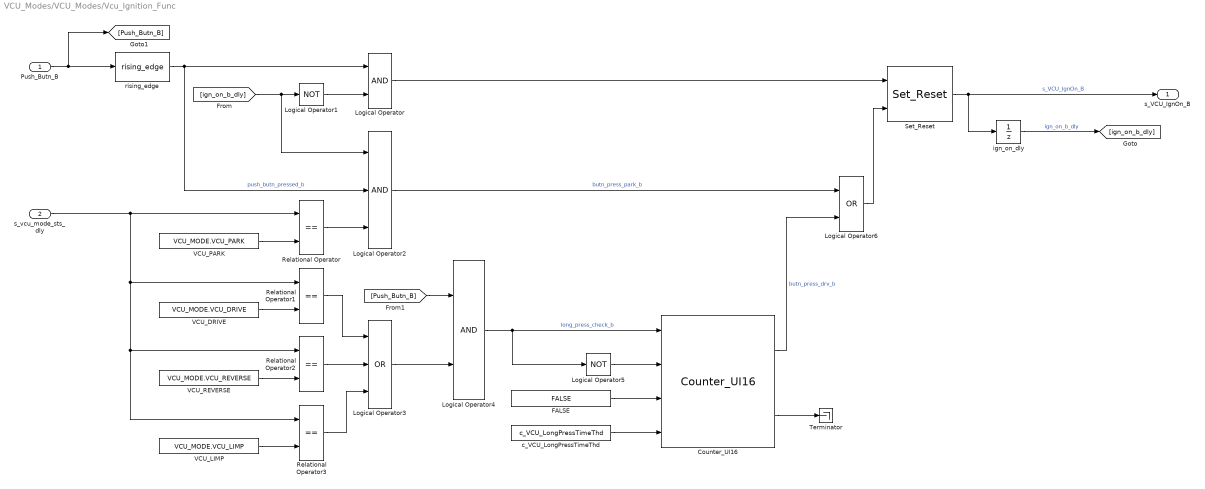
== system VCU_Modes/VCU_Modes/Vcu_Ignition_Func ==
  Push_Butn_B : Inport
  s_vcu_mode_sts_dly : Inport  Port=2
  Counter_UI16 : Sanu_Lib/Counter_UI16  SystemSampleTime=-1  VariantActivationTime=update diagram  EmptyChoice=off  PassThrough=off  PassThroughVariantControl=(default)  EmptyChoiceVariantControl=(default)  AllowFlexibleInterface=on  Latency=0  AutoFrameSizeCalculation=off
  FALSE : Constant  Value=FALSE  OutDataTypeStr=boolean  SampleTime=-1
  Logical Operator : Logic  AllPortsSameDT=off  OutDataTypeStr=boolean
  Logical Operator1 : Logic  Operator=NOT  AllPortsSameDT=off  OutDataTypeStr=boolean
  Logical Operator2 : Logic  Inputs=3  AllPortsSameDT=off  OutDataTypeStr=boolean
  Logical Operator3 : Logic  Operator=OR  Inputs=3  AllPortsSameDT=off  OutDataTypeStr=boolean
  Logical Operator4 : Logic  AllPortsSameDT=off  OutDataTypeStr=boolean
  Logical Operator5 : Logic  Operator=NOT  AllPortsSameDT=off  OutDataTypeStr=boolean
  Logical Operator6 : Logic  Operator=OR  AllPortsSameDT=off  OutDataTypeStr=boolean
  Relational Operator{,1..3} (4 alike) : RelationalOperator  Operator===  OutDataTypeStr=boolean  RndMeth=Simplest  InputSameDT=off
  Set_Reset : Sanu_Lib/Set_Reset  SystemSampleTime=-1  VariantActivationTime=update diagram  EmptyChoice=off  PassThrough=off  PassThroughVariantControl=(default)  EmptyChoiceVariantControl=(default)  AllowFlexibleInterface=on  Latency=0  AutoFrameSizeCalculation=off
  Terminator : Terminator
  VCU_DRIVE : Constant  Value=VCU_MODE.VCU_DRIVE  OutDataTypeStr=Enum: VCU_MODE  SampleTime=-1
  VCU_LIMP : Constant  Value=VCU_MODE.VCU_LIMP  OutDataTypeStr=Enum: VCU_MODE  SampleTime=-1
  VCU_PARK : Constant  Value=VCU_MODE.VCU_PARK  OutDataTypeStr=Enum: VCU_MODE  SampleTime=-1
  VCU_REVERSE : Constant  Value=VCU_MODE.VCU_REVERSE  OutDataTypeStr=Enum: VCU_MODE  SampleTime=-1
  c_VCU_LongPressTimeThd : Constant  Value=c_VCU_LongPressTimeThd  OutDataTypeStr=uint16  SampleTime=-1
  ign_on_dly : UnitDelay  InitialCondition=false  SampleTime=-1  HasFrameUpgradeWarning=on
      settings: AttributesFormatString=Init: %<InitialCondition>
  rising_edge : Sanu_Lib/rising_edge  SystemSampleTime=-1  VariantActivationTime=update diagram  EmptyChoice=off  PassThrough=off  PassThroughVariantControl=(default)  EmptyChoiceVariantControl=(default)  AllowFlexibleInterface=on  Latency=0  AutoFrameSizeCalculation=off
  s_VCU_IgnOn_B : Outport
  wires:
  Push_Butn_B/1 -> [Push_Butn_B], rising_edge/1
  [ign_on_b_dly] -> Logical Operator2/1, Logical Operator1/1
  Logical Operator1/1 -> Logical Operator/2
  Logical Operator/1 -> Set_Reset/1
  VCU_PARK/1 -> Relational Operator/2
  Relational Operator/1 -> Logical Operator2/3
  rising_edge/1 -> Logical Operator/1, Logical Operator2/2  "push_butn_pressed_b"
  s_vcu_mode_sts_dly/1 -> Relational Operator/1, Relational Operator1/1, Relational Operator3/1, Relational Operator2/1
  VCU_DRIVE/1 -> Relational Operator1/2
  VCU_REVERSE/1 -> Relational Operator2/2
  VCU_LIMP/1 -> Relational Operator3/2
  Relational Operator1/1 -> Logical Operator3/1
  Relational Operator2/1 -> Logical Operator3/2
  Relational Operator3/1 -> Logical Operator3/3
  Logical Operator3/1 -> Logical Operator4/2
  [Push_Butn_B] -> Logical Operator4/1
  Logical Operator4/1 -> Logical Operator5/1, Counter_UI16/1  "long_press_check_b"
  Logical Operator5/1 -> Counter_UI16/2
  c_VCU_LongPressTimeThd/1 -> Counter_UI16/4
  FALSE/1 -> Counter_UI16/3
  Counter_UI16/2 -> Terminator/1
  Counter_UI16/1 -> Logical Operator6/2  "butn_press_drv_b"
  Logical Operator2/1 -> Logical Operator6/1  "butn_press_park_b"
  Logical Operator6/1 -> Set_Reset/2
  Set_Reset/1 -> ign_on_dly/1, s_VCU_IgnOn_B/1  "s_VCU_IgnOn_B"
  ign_on_dly/1 -> [ign_on_b_dly]  "ign_on_b_dly"

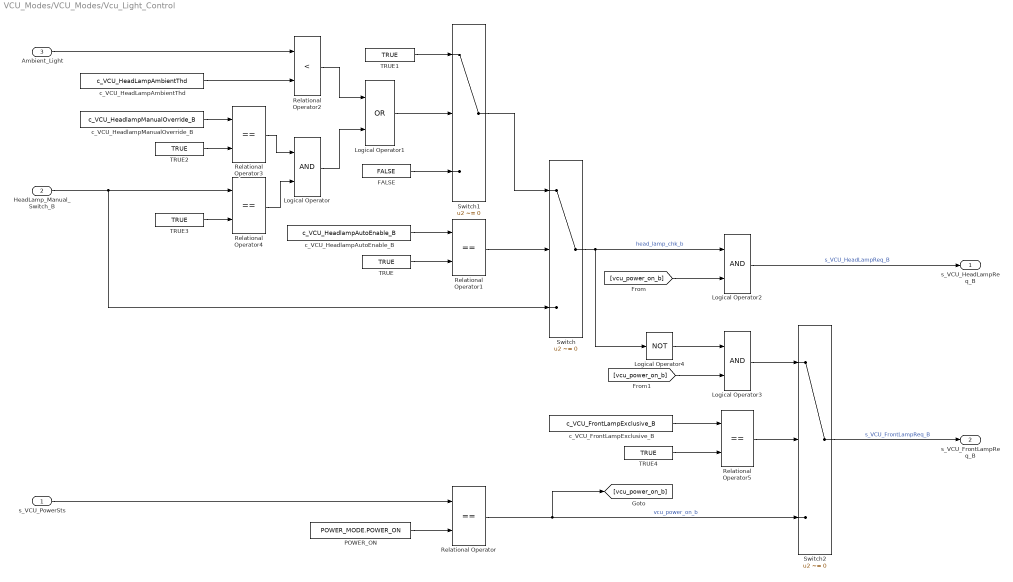
== system VCU_Modes/VCU_Modes/Vcu_Light_Control ==
  s_VCU_PowerSts : Inport
  HeadLamp_Manual_Switch_B : Inport  Port=2
  Ambient_Light : Inport  Port=3
  FALSE : Constant  Value=FALSE  OutDataTypeStr=boolean  SampleTime=-1
  Logical Operator : Logic  AllPortsSameDT=off  OutDataTypeStr=boolean
  Logical Operator1 : Logic  Operator=OR  AllPortsSameDT=off  OutDataTypeStr=boolean
  Logical Operator2 : Logic  AllPortsSameDT=off  OutDataTypeStr=boolean
  Logical Operator3 : Logic  AllPortsSameDT=off  OutDataTypeStr=boolean
  Logical Operator4 : Logic  Operator=NOT  AllPortsSameDT=off  OutDataTypeStr=boolean
  POWER_ON : Constant  Value=POWER_MODE.POWER_ON  OutDataTypeStr=Enum: POWER_MODE  SampleTime=-1
  Relational Operator{,1,3..5} (5 alike) : RelationalOperator  Operator===  OutDataTypeStr=boolean  RndMeth=Simplest  InputSameDT=off
  Relational Operator2 : RelationalOperator  Operator=<  OutDataTypeStr=boolean  RndMeth=Simplest  InputSameDT=off
  Switch : Switch  Criteria=u2 ~= 0  SaturateOnIntegerOverflow=off  InputSameDT=off
  Switch1 : Switch  Criteria=u2 ~= 0  SaturateOnIntegerOverflow=off  InputSameDT=off
  Switch2 : Switch  Criteria=u2 ~= 0  SaturateOnIntegerOverflow=off  InputSameDT=off
  TRUE{,1..4} (5 alike) : Constant  Value=TRUE  OutDataTypeStr=boolean  SampleTime=-1
  c_VCU_FrontLampExclusive_B : Constant  Value=c_VCU_FrontLampExclusive_B  OutDataTypeStr=boolean  SampleTime=-1
  c_VCU_HeadLampAmbientThd : Constant  Value=c_VCU_HeadLampAmbientThd  OutDataTypeStr=uint16  SampleTime=-1
  "c_VCU_HeadlampAutoEnable_B " : Constant  Value=c_VCU_HeadlampAutoEnable_B  OutDataTypeStr=boolean  SampleTime=-1
  "c_VCU_HeadlampManualOverride_B " : Constant  Value=c_VCU_HeadlampManualOverride_B  OutDataTypeStr=boolean  SampleTime=-1
  s_VCU_HeadLampReq_B : Outport
  s_VCU_FrontLampReq_B : Outport  Port=2
  wires:
  s_VCU_PowerSts/1 -> Relational Operator/1
  POWER_ON/1 -> Relational Operator/2
  Switch2/1 -> s_VCU_FrontLampReq_B/1  "s_VCU_FrontLampReq_B"
  Relational Operator/1 -> [vcu_power_on_b], Switch2/3  "vcu_power_on_b"
  HeadLamp_Manual_Switch_B/1 -> Switch/3, Relational Operator4/1
  "c_VCU_HeadlampAutoEnable_B "/1 -> Relational Operator1/1
  Ambient_Light/1 -> Relational Operator2/1
  c_VCU_HeadLampAmbientThd/1 -> Relational Operator2/2
  Relational Operator2/1 -> Logical Operator1/1
  Logical Operator/1 -> Logical Operator1/2
  Logical Operator1/1 -> Switch1/2
  FALSE/1 -> Switch1/3
  Switch1/1 -> Switch/1
  Relational Operator1/1 -> Switch/2
  TRUE/1 -> Relational Operator1/2
  TRUE1/1 -> Switch1/1
  Relational Operator3/1 -> Logical Operator/1
  "c_VCU_HeadlampManualOverride_B "/1 -> Relational Operator3/1
  TRUE2/1 -> Relational Operator3/2
  TRUE3/1 -> Relational Operator4/2
  Relational Operator4/1 -> Logical Operator/2
  TRUE4/1 -> Relational Operator5/2
  c_VCU_FrontLampExclusive_B/1 -> Relational Operator5/1
  Relational Operator5/1 -> Switch2/2
  Switch/1 -> Logical Operator4/1, Logical Operator2/1  "head_lamp_chk_b"
  Logical Operator2/1 -> s_VCU_HeadLampReq_B/1  "s_VCU_HeadLampReq_B"
  Logical Operator3/1 -> Switch2/1
  [vcu_power_on_b] -> Logical Operator2/2
  [vcu_power_on_b] -> Logical Operator3/2
  Logical Operator4/1 -> Logical Operator3/1

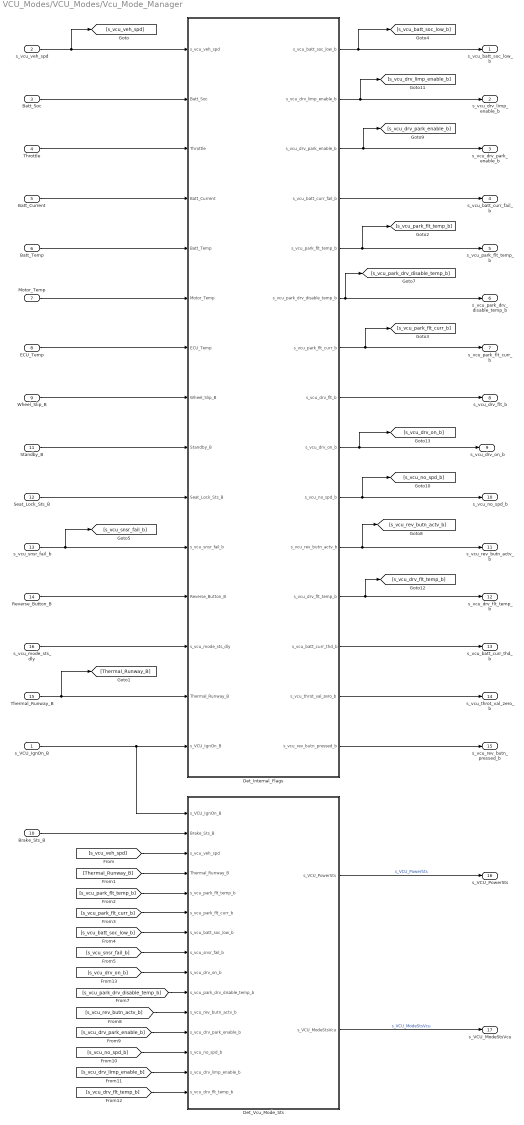
== system VCU_Modes/VCU_Modes/Vcu_Mode_Manager ==
  s_VCU_IgnOn_B : Inport
  s_vcu_veh_spd : Inport  Port=2
  Batt_Soc : Inport  Port=3
  Throttle : Inport  Port=4
  Batt_Current : Inport  Port=5
  Batt_Temp : Inport  Port=6
  Motor_Temp : Inport  Port=7
  ECU_Temp : Inport  Port=8
  Wheel_Slip_B : Inport  Port=9
  Brake_Sts_B : Inport  Port=10
  Standby_B : Inport  Port=11
  Seat_Lock_Sts_B : Inport  Port=12
  s_vcu_snsr_fail_b : Inport  Port=13
  Reverse_Button_B : Inport  Port=14
  Thermal_Runway_B : Inport  Port=15
  s_vcu_mode_sts_dly : Inport  Port=16
  Det_Internal_Flags : Subsystem
  Det_Vcu_Mode_Sts : Subsystem
  s_vcu_batt_soc_low_b : Outport
  s_vcu_drv_limp_enable_b : Outport  Port=2
  s_vcu_drv_park_enable_b : Outport  Port=3
  s_vcu_batt_curr_fail_b : Outport  Port=4
  s_vcu_park_flt_temp_b : Outport  Port=5
  s_vcu_park_drv_disable_temp_b : Outport  Port=6
  s_vcu_park_flt_curr_b : Outport  Port=7
  s_vcu_drv_flt_b : Outport  Port=8
  s_vcu_drv_on_b : Outport  Port=9
  s_vcu_no_spd_b : Outport  Port=10
  s_vcu_rev_butn_actv_b : Outport  Port=11
  s_vcu_drv_flt_temp_b : Outport  Port=12
  s_vcu_batt_curr_thd_b : Outport  Port=13
  s_vcu_throt_val_zero_b : Outport  Port=14
  s_vcu_rev_butn_pressed_b : Outport  Port=15
  s_VCU_PowerSts : Outport  Port=16
  s_VCU_ModeStsVcu : Outport  Port=17
  wires:
  Det_Internal_Flags/8(s_vcu_drv_flt_b) -> s_vcu_drv_flt_b/1
  Motor_Temp/1 -> Det_Internal_Flags/6(Motor_Temp)
  Det_Internal_Flags/9(s_vcu_drv_on_b) -> s_vcu_drv_on_b/1, [s_vcu_drv_on_b]
  Det_Internal_Flags/11(s_vcu_rev_butn_actv_b) -> s_vcu_rev_butn_actv_b/1, [s_vcu_rev_butn_actv_b]
  Wheel_Slip_B/1 -> Det_Internal_Flags/8(Wheel_Slip_B)
  ECU_Temp/1 -> Det_Internal_Flags/7(ECU_Temp)
  Det_Internal_Flags/7(s_vcu_park_flt_curr_b) -> s_vcu_park_flt_curr_b/1, [s_vcu_park_flt_curr_b]
  Standby_B/1 -> Det_Internal_Flags/9(Standby_B)
  Det_Internal_Flags/2(s_vcu_drv_limp_enable_b) -> s_vcu_drv_limp_enable_b/1, [s_vcu_drv_limp_enable_b]
  Seat_Lock_Sts_B/1 -> Det_Internal_Flags/10(Seat_Lock_Sts_B)
  Det_Internal_Flags/1(s_vcu_batt_soc_low_b) -> s_vcu_batt_soc_low_b/1, [s_vcu_batt_soc_low_b]
  s_vcu_snsr_fail_b/1 -> [s_vcu_snsr_fail_b], Det_Internal_Flags/11(s_vcu_snsr_fail_b)
  Det_Internal_Flags/5(s_vcu_park_flt_temp_b) -> s_vcu_park_flt_temp_b/1, [s_vcu_park_flt_temp_b]
  Det_Internal_Flags/4(s_vcu_batt_curr_fail_b) -> s_vcu_batt_curr_fail_b/1
  s_vcu_mode_sts_dly/1 -> Det_Internal_Flags/13(s_vcu_mode_sts_dly)
  Det_Internal_Flags/3(s_vcu_drv_park_enable_b) -> s_vcu_drv_park_enable_b/1, [s_vcu_drv_park_enable_b]
  Reverse_Button_B/1 -> Det_Internal_Flags/12(Reverse_Button_B)
  Det_Internal_Flags/6(s_vcu_park_drv_disable_temp_b) -> s_vcu_park_drv_disable_temp_b/1, [s_vcu_park_drv_disable_temp_b]
  Batt_Current/1 -> Det_Internal_Flags/4(Batt_Current)
  Throttle/1 -> Det_Internal_Flags/3(Throttle)
  Batt_Soc/1 -> Det_Internal_Flags/2(Batt_Soc)
  s_vcu_veh_spd/1 -> [s_vcu_veh_spd], Det_Internal_Flags/1(s_vcu_veh_spd)
  Batt_Temp/1 -> Det_Internal_Flags/5(Batt_Temp)
  s_VCU_IgnOn_B/1 -> Det_Internal_Flags/15(s_VCU_IgnOn_B), Det_Vcu_Mode_Sts/1(s_VCU_IgnOn_B)
  Brake_Sts_B/1 -> Det_Vcu_Mode_Sts/2(Brake_Sts_B)
  Det_Internal_Flags/10(s_vcu_no_spd_b) -> s_vcu_no_spd_b/1, [s_vcu_no_spd_b]
  [s_vcu_veh_spd] -> Det_Vcu_Mode_Sts/3(s_vcu_veh_spd)
  Thermal_Runway_B/1 -> [Thermal_Runway_B], Det_Internal_Flags/14(Thermal_Runway_B)
  [Thermal_Runway_B] -> Det_Vcu_Mode_Sts/4(Thermal_Runway_B)
  [s_vcu_park_flt_temp_b] -> Det_Vcu_Mode_Sts/5(s_vcu_park_flt_temp_b)
  [s_vcu_park_flt_curr_b] -> Det_Vcu_Mode_Sts/6(s_vcu_park_flt_curr_b)
  Det_Vcu_Mode_Sts/1(s_VCU_PowerSts) -> s_VCU_PowerSts/1  "s_VCU_PowerSts"
  Det_Vcu_Mode_Sts/2(s_VCU_ModeStsVcu) -> s_VCU_ModeStsVcu/1  "s_VCU_ModeStsVcu"
  [s_vcu_batt_soc_low_b] -> Det_Vcu_Mode_Sts/7(s_vcu_batt_soc_low_b)
  [s_vcu_snsr_fail_b] -> Det_Vcu_Mode_Sts/8(s_vcu_snsr_fail_b)
  [s_vcu_drv_on_b] -> Det_Vcu_Mode_Sts/9(s_vcu_drv_on_b)
  [s_vcu_park_drv_disable_temp_b] -> Det_Vcu_Mode_Sts/10(s_vcu_park_drv_disable_temp_b)
  [s_vcu_rev_butn_actv_b] -> Det_Vcu_Mode_Sts/11(s_vcu_rev_butn_actv_b)
  [s_vcu_drv_park_enable_b] -> Det_Vcu_Mode_Sts/12(s_vcu_drv_park_enable_b)
  [s_vcu_no_spd_b] -> Det_Vcu_Mode_Sts/13(s_vcu_no_spd_b)
  [s_vcu_drv_limp_enable_b] -> Det_Vcu_Mode_Sts/14(s_vcu_drv_limp_enable_b)
  Det_Internal_Flags/12(s_vcu_drv_flt_temp_b) -> [s_vcu_drv_flt_temp_b], s_vcu_drv_flt_temp_b/1
  Det_Internal_Flags/13(s_vcu_batt_curr_thd_b) -> s_vcu_batt_curr_thd_b/1
  Det_Internal_Flags/14(s_vcu_throt_val_zero_b) -> s_vcu_throt_val_zero_b/1
  [s_vcu_drv_flt_temp_b] -> Det_Vcu_Mode_Sts/15(s_vcu_drv_flt_temp_b)
  Det_Internal_Flags/15(s_vcu_rev_butn_pressed_b) -> s_vcu_rev_butn_pressed_b/1

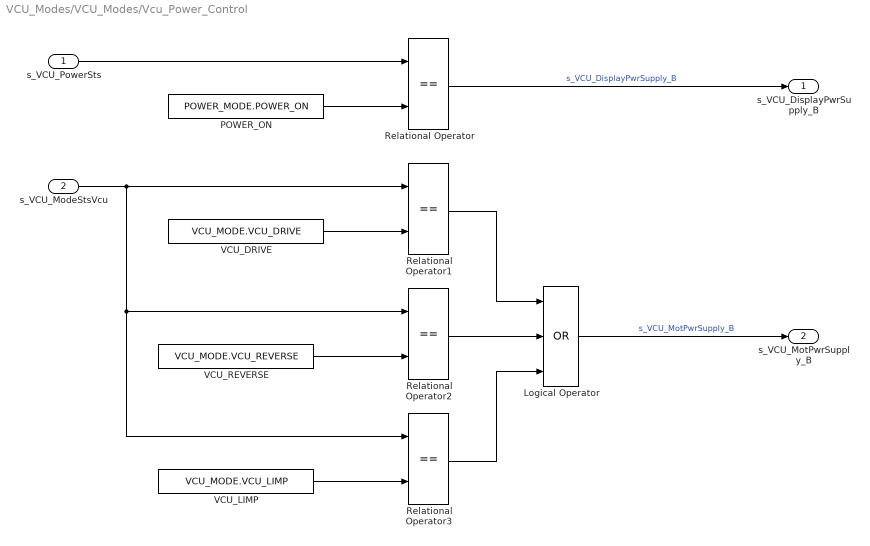
== system VCU_Modes/VCU_Modes/Vcu_Power_Control ==
  s_VCU_PowerSts : Inport
  "s_VCU_ModeStsVcu " : Inport  Port=2
  Logical Operator : Logic  Operator=OR  Inputs=3  AllPortsSameDT=off  OutDataTypeStr=boolean
  POWER_ON : Constant  Value=POWER_MODE.POWER_ON  OutDataTypeStr=Enum: POWER_MODE  SampleTime=-1
  Relational Operator{,1..3} (4 alike) : RelationalOperator  Operator===  OutDataTypeStr=boolean  RndMeth=Simplest  InputSameDT=off
  VCU_DRIVE : Constant  Value=VCU_MODE.VCU_DRIVE  OutDataTypeStr=Enum: VCU_MODE  SampleTime=-1
  VCU_LIMP : Constant  Value=VCU_MODE.VCU_LIMP  OutDataTypeStr=Enum: VCU_MODE  SampleTime=-1
  VCU_REVERSE : Constant  Value=VCU_MODE.VCU_REVERSE  OutDataTypeStr=Enum: VCU_MODE  SampleTime=-1
  s_VCU_DisplayPwrSupply_B : Outport
  s_VCU_MotPwrSupply_B : Outport  Port=2
  wires:
  s_VCU_PowerSts/1 -> Relational Operator/1
  Relational Operator/1 -> s_VCU_DisplayPwrSupply_B/1  "s_VCU_DisplayPwrSupply_B"
  POWER_ON/1 -> Relational Operator/2
  "s_VCU_ModeStsVcu "/1 -> Relational Operator2/1, Relational Operator3/1, Relational Operator1/1
  VCU_DRIVE/1 -> Relational Operator1/2
  VCU_REVERSE/1 -> Relational Operator2/2
  VCU_LIMP/1 -> Relational Operator3/2
  Relational Operator2/1 -> Logical Operator/2
  Relational Operator1/1 -> Logical Operator/1
  Relational Operator3/1 -> Logical Operator/3
  Logical Operator/1 -> s_VCU_MotPwrSupply_B/1  "s_VCU_MotPwrSupply_B"

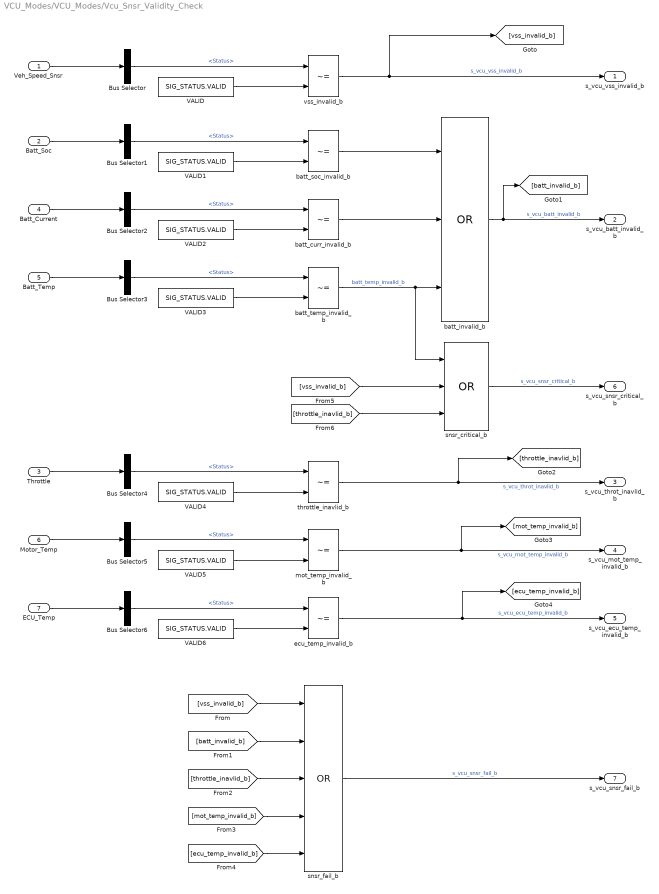
== system VCU_Modes/VCU_Modes/Vcu_Snsr_Validity_Check ==
  Veh_Speed_Snsr : Inport
  Batt_Soc : Inport  Port=2
  Throttle : Inport  Port=3
  Batt_Current : Inport  Port=4
  Batt_Temp : Inport  Port=5
  Motor_Temp : Inport  Port=6
  ECU_Temp : Inport  Port=7
  Bus Selector{,1..6} (7 alike) : BusSelector  OutputSignals=Status
  VALID{,1..6} (7 alike) : Constant  Value=SIG_STATUS.VALID  SampleTime=-1
  batt_curr_invalid_b : RelationalOperator  Operator=~=  OutDataTypeStr=boolean  RndMeth=Simplest  InputSameDT=off
  batt_invalid_b : Logic  Operator=OR  Inputs=3  AllPortsSameDT=off  OutDataTypeStr=boolean
  batt_soc_invalid_b : RelationalOperator  Operator=~=  OutDataTypeStr=boolean  RndMeth=Simplest  InputSameDT=off
  batt_temp_invalid_b : RelationalOperator  Operator=~=  OutDataTypeStr=boolean  RndMeth=Simplest  InputSameDT=off
  ecu_temp_invalid_b : RelationalOperator  Operator=~=  OutDataTypeStr=boolean  RndMeth=Simplest  InputSameDT=off
  mot_temp_invalid_b : RelationalOperator  Operator=~=  OutDataTypeStr=boolean  RndMeth=Simplest  InputSameDT=off
  snsr_critical_b : Logic  Operator=OR  Inputs=3  AllPortsSameDT=off  OutDataTypeStr=boolean
  snsr_fail_b : Logic  Operator=OR  Inputs=5  AllPortsSameDT=off  OutDataTypeStr=boolean
  throttle_inavlid_b : RelationalOperator  Operator=~=  OutDataTypeStr=boolean  RndMeth=Simplest  InputSameDT=off
  vss_invalid_b : RelationalOperator  Operator=~=  OutDataTypeStr=boolean  RndMeth=Simplest  InputSameDT=off
  s_vcu_vss_invalid_b : Outport
  s_vcu_batt_invalid_b : Outport  Port=2
  s_vcu_throt_inavlid_b : Outport  Port=3
  s_vcu_mot_temp_invalid_b : Outport  Port=4
  s_vcu_ecu_temp_invalid_b : Outport  Port=5
  s_vcu_snsr_critical_b : Outport  Port=6
  s_vcu_snsr_fail_b : Outport  Port=7
  wires:
  [ecu_temp_invalid_b] -> snsr_fail_b/5
  [mot_temp_invalid_b] -> snsr_fail_b/4
  [throttle_inavlid_b] -> snsr_fail_b/3
  [batt_invalid_b] -> snsr_fail_b/2
  [vss_invalid_b] -> snsr_fail_b/1
  mot_temp_invalid_b/1 -> s_vcu_mot_temp_invalid_b/1, [mot_temp_invalid_b]  "s_vcu_mot_temp_invalid_b"
  throttle_inavlid_b/1 -> s_vcu_throt_inavlid_b/1, [throttle_inavlid_b]  "s_vcu_throt_inavlid_b"
  ecu_temp_invalid_b/1 -> s_vcu_ecu_temp_invalid_b/1, [ecu_temp_invalid_b]  "s_vcu_ecu_temp_invalid_b"
  Throttle/1 -> Bus Selector4/1
  Motor_Temp/1 -> Bus Selector5/1
  ECU_Temp/1 -> Bus Selector6/1
  VALID4/1 -> throttle_inavlid_b/2
  Bus Selector4/1 -> throttle_inavlid_b/1  "<Status>"
  Bus Selector5/1 -> mot_temp_invalid_b/1  "<Status>"
  VALID5/1 -> mot_temp_invalid_b/2
  VALID6/1 -> ecu_temp_invalid_b/2
  Bus Selector6/1 -> ecu_temp_invalid_b/1  "<Status>"
  batt_invalid_b/1 -> s_vcu_batt_invalid_b/1, [batt_invalid_b]  "s_vcu_batt_invalid_b"
  vss_invalid_b/1 -> s_vcu_vss_invalid_b/1, [vss_invalid_b]  "s_vcu_vss_invalid_b"
  batt_temp_invalid_b/1 -> snsr_critical_b/1, batt_invalid_b/3  "batt_temp_invalid_b"
  batt_curr_invalid_b/1 -> batt_invalid_b/2
  batt_soc_invalid_b/1 -> batt_invalid_b/1
  Batt_Temp/1 -> Bus Selector3/1
  Bus Selector3/1 -> batt_temp_invalid_b/1  "<Status>"
  VALID3/1 -> batt_temp_invalid_b/2
  VALID2/1 -> batt_curr_invalid_b/2
  Bus Selector2/1 -> batt_curr_invalid_b/1  "<Status>"
  Bus Selector1/1 -> batt_soc_invalid_b/1  "<Status>"
  VALID1/1 -> batt_soc_invalid_b/2
  Batt_Current/1 -> Bus Selector2/1
  VALID/1 -> vss_invalid_b/2
  Bus Selector/1 -> vss_invalid_b/1  "<Status>"
  Batt_Soc/1 -> Bus Selector1/1
  Veh_Speed_Snsr/1 -> Bus Selector/1
  [throttle_inavlid_b] -> snsr_critical_b/3
  [vss_invalid_b] -> snsr_critical_b/2
  snsr_critical_b/1 -> s_vcu_snsr_critical_b/1  "s_vcu_snsr_critical_b"
  snsr_fail_b/1 -> s_vcu_snsr_fail_b/1  "s_vcu_snsr_fail_b"
